simulink model "rota"  (R2020b)
settings: Solver=VariableStepAuto  StartTime=0.0  StopTime=100  RelTol=1e-3
undefined symbols (not defined in the file or in its folder): I1, I2, K1, K2
settings Model: Creator=Acer  LastModifiedBy=Acer

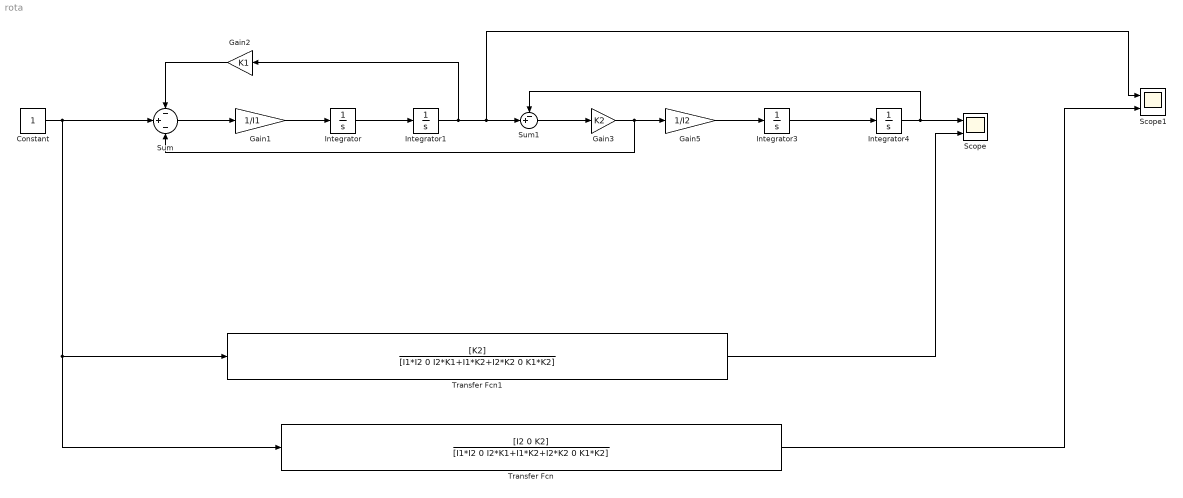
== system rota ==
  Constant : Constant
  Gain1 : Gain  Gain=1/I1
  Gain2 : Gain  Gain=K1
  Gain3 : Gain  Gain=K2
  Gain5 : Gain  Gain=1/I2
  Integrator{,1,3..4} (4 alike) : Integrator
  Scope : Scope  NumInputPorts=2
  Scope1 : Scope  NumInputPorts=2
  Sum : Sum  Inputs=-+-
  Sum1 : Sum  Inputs=-+|
  Transfer Fcn : TransferFcn  Numerator=[I2 0 K2]  Denominator=[I1*I2 0 I2*K1+I1*K2+I2*K2 0 K1*K2]
  Transfer Fcn1 : TransferFcn  Numerator=[K2]  Denominator=[I1*I2 0 I2*K1+I1*K2+I2*K2 0 K1*K2]
  wires:
  Integrator3/1 -> Integrator4/1
  Integrator4/1 -> Sum1/1, Scope/1
  Constant/1 -> Sum/2, Transfer Fcn/1, Transfer Fcn1/1
  Gain5/1 -> Integrator3/1
  Integrator/1 -> Integrator1/1
  Gain2/1 -> Sum/1
  Gain1/1 -> Integrator/1
  Transfer Fcn/1 -> Scope1/2
  Sum/1 -> Gain1/1
  Transfer Fcn1/1 -> Scope/2
  Integrator1/1 -> Gain2/1, Scope1/1, Sum1/2
  Gain3/1 -> Sum/3, Gain5/1
  Sum1/1 -> Gain3/1
